simulink model "brake"  (R2021a)
settings: Solver=VariableStepAuto  StartTime=0.0  StopTime=10.0  RelTol=1e-3
values from neighbouring files (symbols this model uses):
  x0 = X0 - pt    [Final_Control.m]    (also in control.m; control_d.m)
undefined symbols (not defined in the file or in its folder): l0, phi0, theta0, z0
settings Model: Creator=Usuario  LastModifiedBy=Usuario

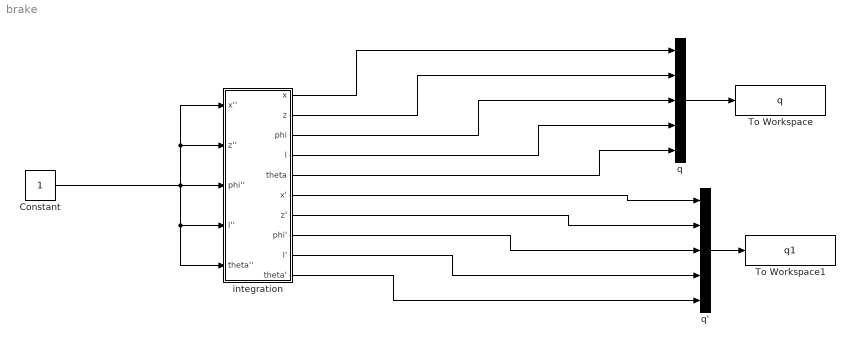
== system brake ==
  Constant : Constant
  To Workspace : ToWorkspace  VariableName=q  SaveFormat=Timeseries  SampleTime=-1
  To Workspace1 : ToWorkspace  VariableName=q1  SaveFormat=Timeseries  SampleTime=-1
  integration : Subsystem
  q : Mux  Inputs=5
  q' : Mux  Inputs=5
  wires:
  q/1 -> To Workspace/1
  q'/1 -> To Workspace1/1
  Constant/1 -> integration/5(theta''), integration/4(l''), integration/1(x''), integration/2(z''), integration/3(phi'')
  integration/1(x) -> q/1
  integration/2(z) -> q/2
  integration/3(phi) -> q/3
  integration/4(l) -> q/4
  integration/5(theta) -> q/5
  integration/6(x') -> q'/1
  integration/7(z') -> q'/2
  integration/8(phi') -> q'/3
  integration/9(l') -> q'/4
  integration/10(theta') -> q'/5

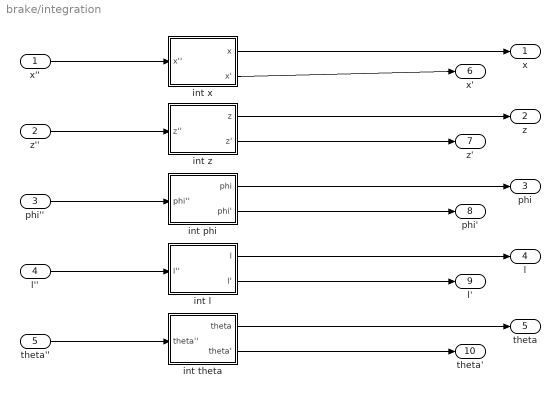
== system brake/integration ==
  x'' : Inport
  z'' : Inport  Port=2
  phi'' : Inport  Port=3
  l'' : Inport  Port=4
  theta'' : Inport  Port=5
  int l : Subsystem
  int phi : Subsystem
  int theta : Subsystem
  int x : Subsystem
  int z : Subsystem
  x : Outport
  z : Outport  Port=2
  phi : Outport  Port=3
  l : Outport  Port=4
  theta : Outport  Port=5
  x' : Outport  Port=6
  z' : Outport  Port=7
  phi' : Outport  Port=8
  l' : Outport  Port=9
  theta' : Outport  Port=10
  wires:
  int l/1(l) -> l/1
  int l/2(l') -> l'/1
  int theta/2(theta') -> theta'/1
  int theta/1(theta) -> theta/1
  int phi/1(phi) -> phi/1
  int x/1(x) -> x/1
  int x/2(x') -> x'/1
  int z/1(z) -> z/1
  int z/2(z') -> z'/1
  int phi/2(phi') -> phi'/1
  phi''/1 -> int phi/1(phi'')
  x''/1 -> int x/1(x'')
  z''/1 -> int z/1(z'')
  l''/1 -> int l/1(l'')
  theta''/1 -> int theta/1(theta'')

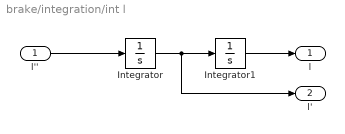
== system brake/integration/int l ==
  l'' : Inport
  Integrator : Integrator
  Integrator1 : Integrator  InitialCondition=l0
  l : Outport
  l' : Outport  Port=2
  wires:
  Integrator/1 -> l'/1, Integrator1/1
  Integrator1/1 -> l/1
  l''/1 -> Integrator/1

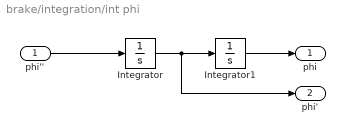
== system brake/integration/int phi ==
  phi'' : Inport
  Integrator : Integrator
  Integrator1 : Integrator  InitialCondition=phi0
  phi : Outport
  phi' : Outport  Port=2
  wires:
  Integrator/1 -> phi'/1, Integrator1/1
  Integrator1/1 -> phi/1
  phi''/1 -> Integrator/1

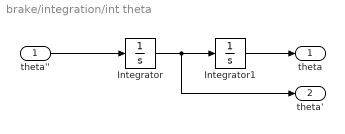
== system brake/integration/int theta ==
  theta'' : Inport
  Integrator : Integrator
  Integrator1 : Integrator  InitialCondition=theta0
  theta : Outport
  theta' : Outport  Port=2
  wires:
  Integrator/1 -> theta'/1, Integrator1/1
  Integrator1/1 -> theta/1
  theta''/1 -> Integrator/1

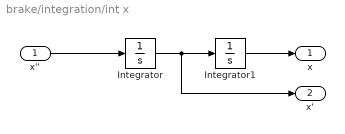
== system brake/integration/int x ==
  x'' : Inport
  Integrator : Integrator
  Integrator1 : Integrator  InitialCondition=x0
  x : Outport
  x' : Outport  Port=2
  wires:
  Integrator/1 -> x'/1, Integrator1/1
  Integrator1/1 -> x/1
  x''/1 -> Integrator/1

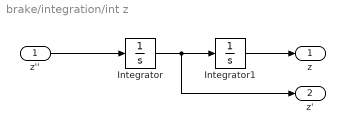
== system brake/integration/int z ==
  z'' : Inport
  Integrator : Integrator
  Integrator1 : Integrator  InitialCondition=z0
  z : Outport
  z' : Outport  Port=2
  wires:
  Integrator/1 -> z'/1, Integrator1/1
  Integrator1/1 -> z/1
  z''/1 -> Integrator/1
